simulink model "SF105A_MotCurrRegVltgLimr"  (R2013b)
settings: Solver=FixedStepDiscrete  SolverMode=SingleTasking  StartTime=0.0  StopTime=1  FixedStep=0.00025  RelTol=1e-3
undefined symbols (not defined in the file): ARCHGLBPRM_2OVERSQRT3_ULS_F32, ARCHGLBPRM_2PI_ULS_F32, BRDGVLTGHILIM_VOLT_F32, ELECGLBPRM_PWMPERDNOMX2_SEC_F32, F32TOU16OVR2PI_ULS_F32, MotCurrRegCfgCurrLoopSecOrderTrfFctEna, MotCurrRegCfgMotRVirtDax, MotCurrRegCfgMotRVirtQax, MotCurrRegVltgLimrCurrLoaScarSlewRate, MotCurrRegVltgLimrDaxAntiWdupCoeff, MotCurrRegVltgLimrDualEcuLoaScarSlewRate, MotCurrRegVltgLimrIvtrLoaScarSlewRate, MotCurrRegVltgLimrMotCurrPredEna, MotCurrRegVltgLimrMotCurrPredTi, MotCurrRegVltgLimrMotCurrQaxRefMdfnRplEna, MotCurrRegVltgLimrMotVltgBrdgFilEna, MotCurrRegVltgLimrMotVltgDaxIntglHiLim, MotCurrRegVltgLimrMotVltgDaxIntglLoLim, MotCurrRegVltgLimrMotVltgQaxFfFilEna, MotCurrRegVltgLimrMotVltgQaxIntglHiLim, MotCurrRegVltgLimrMotVltgQaxIntglLoLim, MotCurrRegVltgLimrQaxAntiWdupCoeff, MotCurrRegVltgLimrQaxAntiWdupScagDi, MotRefMdlFbCtrlDi, MotRefMdlIvtrDeadTiBrdgVltgSca, SysSt1, ZERO_VOLT_F32
libraries: NxtrLim x15, Fil x4, simulink x3, NxtrMax x2, NxtrMin x2
(part 1 of 5)
settings Model: Creator=qzwc4r  LastModifiedBy=DZ1YRM
settings SolverCC: AutoInsertRateTranBlk=on  InsertRTBMode=Always
settings DataIOCC: LimitDataPoints=off  SaveFormat=Structure  ReturnWorkspaceOutputs=on
settings OptimizationCC: BlockReduction=off  InlineParams=on  ZeroExternalMemoryAtStartup=off  ZeroInternalMemoryAtStartup=off  OptimizeModelRefInitCode=on  LifeSpan=1
settings DebuggingCC: SignalInfNanChecking=error  SignalRangeChecking=warning  UnderspecifiedInitializationDetection=Simplified  SolverPrmCheckMsg=error  InheritedTsInSrcMsg=error  DiscreteInheritContinuousMsg=error  SingleTaskRateTransMsg=error  TasksWithSamePriorityMsg=error  SigSpecEnsureSampleTimeMsg=error  CheckMatrixSingularityMsg=error  ParameterUnderflowMsg=error  ParameterPrecisionLossMsg=error  ParameterTunabilityLossMsg=error  FixptConstUnderflowMsg=warning  FixptConstOverflowMsg=warning  VectorMatrixConversionMsg=error  SignalLabelMismatchMsg=error  UnconnectedInputMsg=error  UnconnectedOutputMsg=error  UnconnectedLineMsg=error  SFcnCompatibilityMsg=error  UniqueDataStoreMsg=warning  BusObjectLabelMismatch=error  RootOutportRequireBusObject=error  AssertControl=DisableAll  ModelReferenceIOMsg=error  ModelReferenceVersionMismatchMessage=warning  ModelReferenceIOMismatchMessage=error  ModelReferenceCSMismatchMessage=warning  ModelReferenceDataLoggingMessage=error  StateNameClashWarn=warning  StrictBusMsg=ErrorOnBusTreatedAsVector  NonBusSignalsTreatedAsBus=error  SFUnexpectedBacktrackingDiag=error  SFInvalidInputDataAccessInChartInitDiag=error  SFNoUnconditionalDefaultTransitionDiag=error  SFTransitionOutsideNaturalParentDiag=error  SFUnconditionalTransitionShadowingDiag=error  SFUndirectedBroadcastEventsDiag=error
settings ModelReferenceCC: ModelReferenceNumInstancesAllowed=Single
settings RTWCC: SystemTargetFile=autosar.tlc  GenCodeOnly=on  TemplateMakefile=ert_default_tmf  Description=AUTOSAR  GenerateReport=on  ProcessScript=autosar_make_rtw_hook  LaunchReport=on
settings CodeAppCC: GenerateComments=off  IgnoreCustomStorageClasses=off  CustomSymbolStrType=$N$R$M  CustomSymbolStrBlkIO=$N$M  SimulinkBlockComments=off
settings STFCustomTargetCC: ParMdlRefBuildCompliant=on  CompOptLevelCompliant=on  IncludeMdlTerminateFcn=off  CombineOutputUpdateFcns=on  SuppressErrorStatus=on  ERTFirstTimeCompliant=on  ERTCustomFileBanners=on  SupportNonFinite=off  SupportComplex=off  SupportContinuousTime=off  SupportNonInlinedSFcns=off  MATLABClassNameForMDSCustomization=Simulink.SoftwareTarget.ERTCustomization  AutosarCompliant=on  GRTInterface=off  SystemTargetFile=autosar.tlc
settings ERTTargetCC: CodeReplacementLibrary=ANSI_C  ConcurrentExecutionCompliant=off  IncludeMdlTerminateFcn=off  SuppressErrorStatus=on  SupportNonFinite=off  SupportComplex=off  ModelStepFunctionPrototypeControlCompliant=off  CPPClassGenCompliant=off  AutosarCompliant=on  InlinedParameterPlacement=NonHierarchical  ERTCustomFileTemplate=example_file_process.tlc  EnableUserReplacementTypes=on

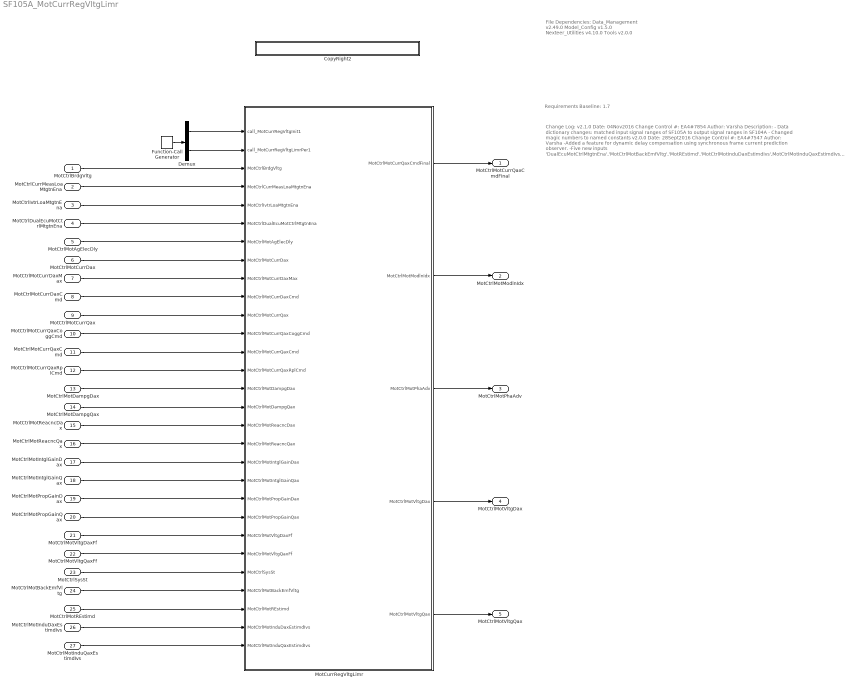
== system SF105A_MotCurrRegVltgLimr ==
  note: File Dependencies:
      |
      | Data_Management v2.49.0
      | Model_Config v1.5.0
      | Nexteer_Utilities v4.10.0
      | Tools v2.0.0
  note: Requirements Baseline: 1.7
  note: Change Log:
      |
      | v2.1.0
      | Date: 04Nov2016
      | Change Control #: EA4#7854
      | Author: Varsha
      | Description:
      | - Data dictionary changes: matched input signal ranges of SF105A to output signal ranges in SF104A
      | - Changed magic numbers to named constants
      |
      |
      | v2.0.0
      | Date: 28Sept2016
      | Change Control #: EA4#7547
      | Author: Varsha
      | -Added a feature for dynamic delay compensation using synchronous frame current prediction observer.
      | -Five new inputs 'DualEcuMotCtrlMtgtnEna','MotCtrlMotBackEmfVltg','MotREstimd','MotCtrlMotInduDaxEstimdIvs',MotCtrlMotInduQaxEstimdIvs
      | have been added to model and data dictionary.
      | -Two new calibrations 'MotCurrRegVltgLimrMotCurrPredEna','MotCurrRegVltgLimrMotCurrPredTi' have been added.
      | -A new constant 'ARCHGLBPRM_2OVERSQRT3_ULS_F32' has been added.
      | -Two per-instance memory blocks 'MotCtrlMotVltgQaxPrev' and 'MotCtrlMotVltgDaxPrev' have been added
      | -Updated design for switching to feedforward control operation during application faulted conditions where single ECU is operational
      |
      | v1.8.0
      | Date: 13Sep2016
      | Change Control #: EA4#7472
      | Author: Siva
      | Description:
      | - Used latest Low Pass filter Initialization blocks.
      |
      | v1.7.0
      | Date: 26Aug2016
      | Change Control #: EA4#7221
      | Author: Siva
      | Description:
      | - Updated Data type conversion block used for calculating Phase Advance from "f32 to u0p16" to "f32 to u16p0"
      |   as the value is converted to "u0p16" upfront using "F32TOU16OVR2PI_ULS_F32" constant.
      |
      |
      | v1.6.0
      | Date: 15Aug2016
      | Change Control #: EA4#6632
      | Author: Siva
      | Description:
      | - Two new constants 'MOTVLTGDQAXLOLIM_VOLT_F32' & 'MOTVLTGDQAXHILIM_VOLT_F32' have been added to
      |   model and Data Dictionary with values -26.5V and +26.5 V respectively for range limiting 'MotCtrlMotVltgDax'
      |   and 'MotCtrlMotVltgQax'.
      | - Two new constants 'PHAADVLOLIM_MOTREV_F32' & 'PHAADVHILIM_MOTREV_F32' have been added to
      |   model and Data Dictionary with values 0 and 65535 respectively for range limiting 'Phase Advance' floating point value.
      | - Updated 'F32TOU16OVR2PI_ULS_F32' constant Value to '10430.21921' instead of '10430.194'.
      | - Removed Saturation limits for 'MotCtrlMotPhaAdv' output signal and added a new Data Type conversion block to
      |   convert float value to u0p16 value.
      | - Removed 'MOTPHAADVHILIM_MOTREV_U0P16' & 'MOTPHAADVLOLIM_MOTREV_U0P16' from Data Dictionary.
      |
      |
      | v1.5.1
      | Date: 29April2016
      | Change Control #: EA4#5367
      | Author: Siva
      | Description:
      | - HIghlighted only those blocks related to v1.5.0.
      |
      |
      | v1.5.0
      | Date: 29April2016
      | Change Control #: EA4#5367
      | Author: Siva
      | Description:
      | - Input signal name changed from 'MotCtrlMotCurrLoaMtgtnEna' to 'MotCtrlCurrMeasLoaMtgtnEna'.
      | - Ranges of calibrations 'MotCurrRegVltgLimrDaxAntiWdupCoeff ' and 'MotCurrRegVltgLimrQaxAntiWdupCoeff'
      |    were updated to -1 & 1 instead of -25 & 25.
      |
      |
      | v1.4.0
      | Date: 04April2015
      | Change Control #: EA4#4493
      | Author: Fei Yuan
      | Description:
      | - Add selectable location for multiply of q axis inverse ratio (multiply by Iq reference , or
      |   multiply by the summation of the Iq reference and Iq ripple and Iq cogging signals).
      | - Add signal range limit on integrator state viriables for q and d axis paths.
      | - Add singal range limit on current reference command per defined signal ranges.
      | - Add signed calibratable integrator state vairable limits.
      |
      | v1.3.0
      | Date: 20November2015
      | Change Control #: EA4#2392
      | Author: Fei Yuan
      | Description:
      | - Add range limiters to outputs
      | - Update the Dependencies in the Data Dict
      | - Correct some keywords based on the keyword list.
      |
      | v1.2.0
      | Date: 05June2015
      | Change Control #: EA4#630
      | DRW: P. Lefler
      | Description:
      | - Fixes to calibration names and data types in DataDict file and Dependencies file.
      |
      | v1.1.0
      | Date: 26May2015
      | Change Control #: EA4#630
      | DRW: P. Lefler
      | Description:
      | - Changes for algorithm optimization, output datatype change, and added requirements links
      |
      | v1.0.0
      | Date: 07May2015
      | Change Control #: EA4#297
      | DRW: P. Lefler
      | Description:
      | - Initial Release
  MotCtrlBrdgVltg : Inport  RequirementInfo={} %GIDa_8e46ce2a_919a_4506_8698_295a99460b12
  MotCtrlCurrMeasLoaMtgtnEna : Inport  RequirementInfo={} %GIDa_af8bb34f_046c_46e7_bd5e_44b54be0502c  Port=2
  MotCtrlIvtrLoaMtgtnEna : Inport  RequirementInfo={} %GIDa_3adfcd90_572b_4e35_8cfd_3c676c239ace  Port=3
  MotCtrlDualEcuMotCtrlMtgtnEna : Inport  RequirementInfo={} %GIDa_4618ed0f_79cf_46df_8a31_52c1690ffb8d  Port=4
  MotCtrlMotAgElecDly : Inport  RequirementInfo={} %GIDa_d64dbb74_7a6c_48e8_b5fd_fb09433ca9f0  Port=5
  MotCtrlMotCurrDax : Inport  RequirementInfo={} %GIDa_e7d34867_bb71_42aa_ae81_73d704cf4016  Port=6
  MotCtrlMotCurrDaxMax : Inport  RequirementInfo={} %GIDa_95b74bd1_5092_49ca_9d39_f9500bf46caa  Port=7
  MotCtrlMotCurrDaxCmd : Inport  RequirementInfo={} %GIDa_68535612_aa98_4b73_9e8e_7c7f66964449  Port=8
  MotCtrlMotCurrQax : Inport  RequirementInfo={} %GIDa_c3d95f7e_4c05_48b0_9da3_bf75894c8661  Port=9
  MotCtrlMotCurrQaxCoggCmd : Inport  RequirementInfo={} %GIDa_d050ecd7_013f_4c96_959a_36eb92ce70ab  Port=10
  MotCtrlMotCurrQaxCmd : Inport  RequirementInfo={} %GIDa_168a24af_4211_4955_a405_77a28ee6b1d8  Port=11
  MotCtrlMotCurrQaxRplCmd : Inport  RequirementInfo={} %GIDa_80f96bb1_811c_4e5c_9c99_d0a2b6d1b546  Port=12
  MotCtrlMotDampgDax : Inport  RequirementInfo={} %GIDa_b4263008_b2fe_479b_ab1a_58326cb85cc1  Port=13
  MotCtrlMotDampgQax : Inport  RequirementInfo={} %GIDa_a343ed71_2ec5_45b3_affe_06b72ae41368  Port=14
  MotCtrlMotReacncDax : Inport  RequirementInfo={} %GIDa_7ae76b1f_2e5a_4874_a1b1_4f7855b8eb50  Port=15
  MotCtrlMotReacncQax : Inport  RequirementInfo={} %GIDa_449f7c36_82cf_4545_8870_73d8e079324d  Port=16
  MotCtrlMotIntglGainDax : Inport  RequirementInfo={} %GIDa_cacd28ef_1570_42d0_8667_de1d5331061d  Port=17
  MotCtrlMotIntglGainQax : Inport  RequirementInfo={} %GIDa_7b09e5f0_cde6_4194_ac39_427519b5ea3c  Port=18
  MotCtrlMotPropGainDax : Inport  RequirementInfo={} %GIDa_722006e4_8def_4c05_955c_20c680c4187a  Port=19
  MotCtrlMotPropGainQax : Inport  RequirementInfo={} %GIDa_be3d4734_242e_476b_ad0b_e25551c24b0a  Port=20
  MotCtrlMotVltgDaxFf : Inport  RequirementInfo={} %GIDa_4efd4844_8ea8_4406_ae94_9804efa9585d  Port=21
  MotCtrlMotVltgQaxFf : Inport  RequirementInfo={} %GIDa_ea442c22_c1cc_4f4a_ada8_81dc7a709cab  Port=22
  MotCtrlSysSt : Inport  RequirementInfo={} %GIDa_be26f1e0_3c0f_4120_aff8_be82e7f083a9  Port=23  OutDataTypeStr=Enum: SysSt1
  MotCtrlMotBackEmfVltg : Inport  RequirementInfo={} %GIDa_f2f564dd_6c3b_46de_9e0e_fc636de52404  Port=24
  MotCtrlMotREstimd : Inport  RequirementInfo={} %GIDa_073120b6_1808_4f14_9c51_29be78d8addc  Port=25
  MotCtrlMotInduDaxEstimdIvs : Inport  RequirementInfo={} %GIDa_a3f48710_1a7a_486c_93c5_3361410e9b98  Port=26
  MotCtrlMotInduQaxEstimdIvs : Inport  RequirementInfo={} %GIDa_79e37907_edf5_439e_bcd8_a58d2ffa50f0  Port=27
  CopyRight2 : Subsystem  Description=|  mask(Copyright Information){none=on}
      | Copyright info block.                                               
      |                                                                     
      | Place copyright information at the top of every subsystem in design.
      mask prompts: none "No parameters"
      mask help: Place copyright information at the top of every subsystem in design.
      mask Display:
      | NxtrConf = 'Nexteer Confidential';
      | 
      | sys = bdroot; %handle for the current model ("system")
      | first = get_param(sys,'Created');
      | if(isempty(first))
      |     first = datestr(now,'yyyy');
      | else
      |     first = first(end-3:end);  %year is last four digits
      | end
      | 
      | last = get_param(sys,'LastModifiedDate');
      | if isempty(last)
      |     last = datestr(now,'yyyy');
      | else
      |     last = last(end-3:end);
      | end
      | 
      | if strcmp(first,last)
      |     fprintf('%s -- Copyright %s Nexteer',NxtrConf,first)
      | else
      |     fprintf('%s -- %s%s- %s Nexteer',NxtrConf,char(169),first,last)
      | end
  Demux : Demux  RequirementInfo={} %GIDa_92189e2f_23ba_494e_b896_c9965fe7d6cd  Outputs=2
  Function-Call Generator : simulink/Ports & Subsystems/Function-Call Generator  RequirementInfo={} %GIDa_d141ba28_1e0a_463b_8f2d_81283afd4db2  sample_time=0.00025  numberOfIterations=1
  MotCurrRegVltgLimr : Subsystem  RequirementInfo={} %GIDa_4642b19e_a30e_4e3c_ab8d_d9e3c3d7ba7b
  MotCtrlMotCurrQaxCmdFinal : Outport  RequirementInfo={} %GIDa_781c28aa_2acd_4b18_9286_344174e8cff2
  MotCtrlMotModlnIdx : Outport  RequirementInfo={} %GIDa_fa51f03d_b9dc_4a13_83b1_4b78852e742e  Port=2
  MotCtrlMotPhaAdv : Outport  RequirementInfo={} %GIDa_ace5b006_310e_4410_94f4_88e59214d43e  Port=3
  MotCtrlMotVltgDax : Outport  RequirementInfo={} %GIDa_04c00acb_66a3_42fd_8198_77a8e17ba56b  Port=4
  MotCtrlMotVltgQax : Outport  RequirementInfo={} %GIDa_039e9d87_d2c8_4e76_ac69_f28813825f03  Port=5
  wires:
  Function-Call Generator/1 -> Demux/1
  Demux/2 -> MotCurrRegVltgLimr/2(call_MotCurrRegVltgLimrPer1)
  Demux/1 -> MotCurrRegVltgLimr/1(call_MotCurrRegVltgInit1)
  MotCtrlBrdgVltg/1 -> MotCurrRegVltgLimr/3(MotCtrlBrdgVltg)
  MotCtrlCurrMeasLoaMtgtnEna/1 -> MotCurrRegVltgLimr/4(MotCtrlCurrMeasLoaMtgtnEna)
  MotCtrlIvtrLoaMtgtnEna/1 -> MotCurrRegVltgLimr/5(MotCtrlIvtrLoaMtgtnEna)
  MotCtrlMotAgElecDly/1 -> MotCurrRegVltgLimr/7(MotCtrlMotAgElecDly)
  MotCtrlMotCurrDax/1 -> MotCurrRegVltgLimr/8(MotCtrlMotCurrDax)
  MotCtrlMotCurrDaxMax/1 -> MotCurrRegVltgLimr/9(MotCtrlMotCurrDaxMax)
  MotCtrlMotCurrDaxCmd/1 -> MotCurrRegVltgLimr/10(MotCtrlMotCurrDaxCmd)
  MotCtrlMotCurrQax/1 -> MotCurrRegVltgLimr/11(MotCtrlMotCurrQax)
  MotCtrlMotCurrQaxCoggCmd/1 -> MotCurrRegVltgLimr/12(MotCtrlMotCurrQaxCoggCmd)
  MotCtrlMotCurrQaxCmd/1 -> MotCurrRegVltgLimr/13(MotCtrlMotCurrQaxCmd)
  MotCtrlMotCurrQaxRplCmd/1 -> MotCurrRegVltgLimr/14(MotCtrlMotCurrQaxRplCmd)
  MotCtrlMotDampgDax/1 -> MotCurrRegVltgLimr/15(MotCtrlMotDampgDax)
  MotCtrlMotDampgQax/1 -> MotCurrRegVltgLimr/16(MotCtrlMotDampgQax)
  MotCtrlMotReacncDax/1 -> MotCurrRegVltgLimr/17(MotCtrlMotReacncDax)
  MotCtrlMotReacncQax/1 -> MotCurrRegVltgLimr/18(MotCtrlMotReacncQax)
  MotCtrlMotIntglGainDax/1 -> MotCurrRegVltgLimr/19(MotCtrlMotIntglGainDax)
  MotCtrlMotIntglGainQax/1 -> MotCurrRegVltgLimr/20(MotCtrlMotIntglGainQax)
  MotCtrlMotPropGainDax/1 -> MotCurrRegVltgLimr/21(MotCtrlMotPropGainDax)
  MotCtrlMotPropGainQax/1 -> MotCurrRegVltgLimr/22(MotCtrlMotPropGainQax)
  MotCtrlMotVltgDaxFf/1 -> MotCurrRegVltgLimr/23(MotCtrlMotVltgDaxFf)
  MotCtrlMotVltgQaxFf/1 -> MotCurrRegVltgLimr/24(MotCtrlMotVltgQaxFf)
  MotCtrlSysSt/1 -> MotCurrRegVltgLimr/25(MotCtrlSysSt)
  MotCurrRegVltgLimr/2(MotCtrlMotModlnIdx) -> MotCtrlMotModlnIdx/1
  MotCurrRegVltgLimr/3(MotCtrlMotPhaAdv) -> MotCtrlMotPhaAdv/1
  MotCurrRegVltgLimr/1(MotCtrlMotCurrQaxCmdFinal) -> MotCtrlMotCurrQaxCmdFinal/1
  MotCurrRegVltgLimr/4(MotCtrlMotVltgDax) -> MotCtrlMotVltgDax/1
  MotCurrRegVltgLimr/5(MotCtrlMotVltgQax) -> MotCtrlMotVltgQax/1
  MotCtrlMotBackEmfVltg/1 -> MotCurrRegVltgLimr/26(MotCtrlMotBackEmfVltg)
  MotCtrlMotREstimd/1 -> MotCurrRegVltgLimr/27(MotCtrlMotREstimd)
  MotCtrlMotInduDaxEstimdIvs/1 -> MotCurrRegVltgLimr/28(MotCtrlMotInduDaxEstimdIvs)
  MotCtrlMotInduQaxEstimdIvs/1 -> MotCurrRegVltgLimr/29(MotCtrlMotInduQaxEstimdIvs)
  MotCtrlDualEcuMotCtrlMtgtnEna/1 -> MotCurrRegVltgLimr/6(MotCtrlDualEcuMotCtrlMtgtnEna)

== system SF105A_MotCurrRegVltgLimr/CopyRight2 ==

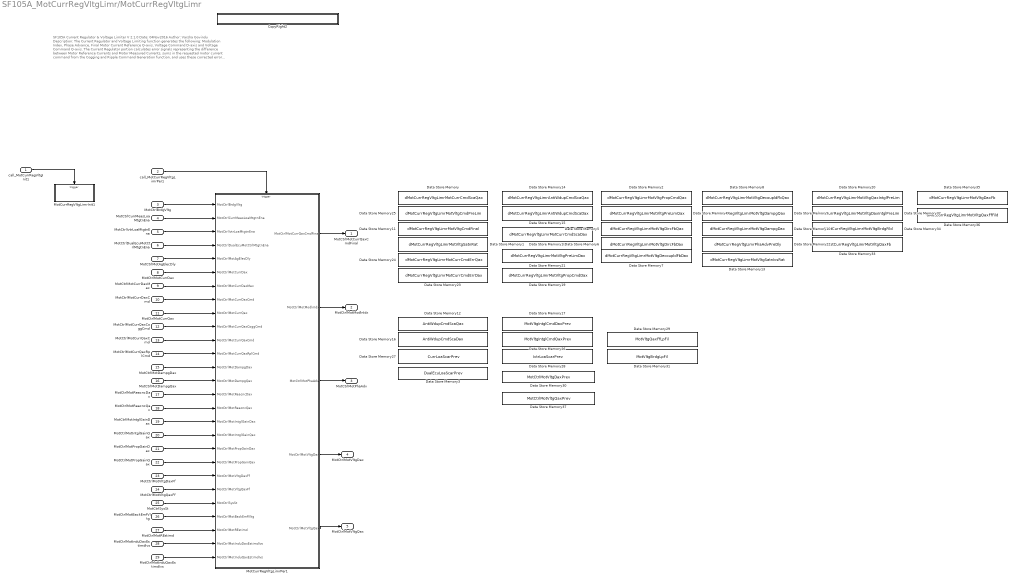
== system SF105A_MotCurrRegVltgLimr/MotCurrRegVltgLimr ==
  note: SF105A Current Regulator & Voltage Limiter
      | V 2.1.0
      | Date: 04Nov2016
      | Author: Varsha Govindu
      | Description: The Current Regulator and Voltage Limiting function generates the following: Modulation Index, Phase Advance, Final Motor Current Reference Q-axis,
      | Voltage Command D-axis and Voltage Command Q-axis.
      | The Current Regulator portion calculates error signals representing the difference between Motor Reference Currents and Motor Measured Currents, sums in the
      | requested motor current command from the Cogging and Ripple Command Generation function, and uses these corrected error signals modified by proportional and
      | integral gains to generate a portion of the voltage command to the motor.  The Current Regulator also applies separate gains to the measured motor currents to
      | generate an additional portion of the voltage command.  The Feedforward Voltages from the Motor Reference model are added to the other two portions to generate
      | the total requested motor voltage command.
      | The Voltage Limiting portion of the function compares the total requested motor voltage command to the total voltage available at the inverter, and implements a limiting
      | and reference command correcting function in order to prevent windup of Current Regulator states and improve reference command tracking.
  call_MotCurrRegVltgInit1 : Inport
  call_MotCurrRegVltgLimrPer1 : Inport  Port=2
  MotCtrlBrdgVltg : Inport  RequirementInfo={'linktype_rmi_doors' '0000bb44 (/E-STEER Core/SubSystem Specifications/Application Functions/SF99/SF105A Current Regulator and Voltage Limiter)' '#SF105A_58' 'true' 'REQ: SF105A_58' '' ; 'linktype_rmi_doors' '0000bb44 (/E-STEER Core/SubSystem Specifications/Application Functions/SF99/SF105A Current Regulator and Voltage Limiter)' '#SF105A_166' 'true' 'REQ: SF105A_166' '' } %GIDa_606dfb72_cb0e_4bf4_a448_cf2d667aea26  Port=3
  MotCtrlCurrMeasLoaMtgtnEna : Inport  RequirementInfo={'linktype_rmi_doors' '0000bb44 (/E-STEER Core/SubSystem Specifications/Application Functions/SF99/SF105A Current Regulator and Voltage Limiter)' '#SF105A_59' 'true' 'REQ: SF105A_59' '' ; 'linktype_rmi_doors' '0000bb44 (/E-STEER Core/SubSystem Specifications/Application Functions/SF99/SF105A Current Regulator and Voltage Limiter)' '#SF105A_168' 'true' 'REQ: SF105A_168' '' } %GIDa_d06f39e9_eb60_46fa_8d46_638325da2097  Port=4
  MotCtrlIvtrLoaMtgtnEna : Inport  RequirementInfo={'linktype_rmi_doors' '0000bb44 (/E-STEER Core/SubSystem Specifications/Application Functions/SF99/SF105A Current Regulator and Voltage Limiter)' '#SF105A_153' 'true' 'REQ: SF105A_153' '' ; 'linktype_rmi_doors' '0000bb44 (/E-STEER Core/SubSystem Specifications/Application Functions/SF99/SF105A Current Regulator and Voltage Limiter)' '#SF105A_168' 'true' 'REQ: SF105A_168' '' } %GIDa_81420cc2_8e05_4f74_9716_a5648030ffcb  Port=5
  MotCtrlDualEcuMotCtrlMtgtnEna : Inport  RequirementInfo={'linktype_rmi_doors' '0000bb44 (/E-STEER Core/SubSystem Specifications/Application Functions/SF99/SF105A Current Regulator and Voltage Limiter)' '#SF105A_199' 'true' 'REQ: SF105A_199' '' } %GIDa_f8a239b4_df34_4f4d_ae99_1298116ecc14  Port=6
  MotCtrlMotAgElecDly : Inport  RequirementInfo={'linktype_rmi_doors' '0000bb44 (/E-STEER Core/SubSystem Specifications/Application Functions/SF99/SF105A Current Regulator and Voltage Limiter)' '#SF105A_46' 'true' 'REQ: SF105A_46' '' } %GIDa_86188211_fab5_49f2_9b91_c05f705e3c63  Port=7
  MotCtrlMotCurrDax : Inport  RequirementInfo={'linktype_rmi_doors' '0000bb44 (/E-STEER Core/SubSystem Specifications/Application Functions/SF99/SF105A Current Regulator and Voltage Limiter)' '#SF105A_57' 'true' 'REQ: SF105A_57' '' } %GIDa_0b9d98be_f12b_4977_b4e0_ba90ca28ad52  Port=8
  MotCtrlMotCurrDaxMax : Inport  RequirementInfo={'linktype_rmi_doors' '0000bb44 (/E-STEER Core/SubSystem Specifications/Application Functions/SF99/SF105A Current Regulator and Voltage Limiter)' '#SF105A_53' 'true' 'REQ: SF105A_53' '' } %GIDa_6012c004_0bcf_42a3_ab54_1ad4e16fdcd8  Port=9
  MotCtrlMotCurrDaxCmd : Inport  RequirementInfo={'linktype_rmi_doors' '0000bb44 (/E-STEER Core/SubSystem Specifications/Application Functions/SF99/SF105A Current Regulator and Voltage Limiter)' '#SF105A_38' 'true' 'REQ: SF105A_38' '' } %GIDa_3c8cfcc2_1716_43e3_a5f4_74f0cc4785f3  Port=10
  MotCtrlMotCurrQax : Inport  RequirementInfo={'linktype_rmi_doors' '0000bb44 (/E-STEER Core/SubSystem Specifications/Application Functions/SF99/SF105A Current Regulator and Voltage Limiter)' '#SF105A_56' 'true' 'REQ: SF105A_56' '' } %GIDa_f2105923_8b5d_4c38_b5d7_d8944874b87d  Port=11
  MotCtrlMotCurrQaxCoggCmd : Inport  RequirementInfo={'linktype_rmi_doors' '0000bb44 (/E-STEER Core/SubSystem Specifications/Application Functions/SF99/SF105A Current Regulator and Voltage Limiter)' '#SF105A_47' 'true' 'REQ: SF105A_47' '' } %GIDa_5eb15454_dd57_4a66_beac_3c42276a2f51  Port=12
  MotCtrlMotCurrQaxCmd : Inport  RequirementInfo={'linktype_rmi_doors' '0000bb44 (/E-STEER Core/SubSystem Specifications/Application Functions/SF99/SF105A Current Regulator and Voltage Limiter)' '#SF105A_27' 'true' 'REQ: SF105A_27' '' } %GIDa_00ed98c3_1b47_4f14_b89e_6bdb9443e2b5  Port=13
  MotCtrlMotCurrQaxRplCmd : Inport  RequirementInfo={'linktype_rmi_doors' '0000bb44 (/E-STEER Core/SubSystem Specifications/Application Functions/SF99/SF105A Current Regulator and Voltage Limiter)' '#SF105A_48' 'true' 'REQ: SF105A_48' '' } %GIDa_164b68d2_17d4_417d_9d13_ce78fec31a24  Port=14
  MotCtrlMotDampgDax : Inport  RequirementInfo={'linktype_rmi_doors' '0000bb44 (/E-STEER Core/SubSystem Specifications/Application Functions/SF99/SF105A Current Regulator and Voltage Limiter)' '#SF105A_51' 'true' 'REQ: SF105A_51' '' } %GIDa_d80b900b_5b17_49e7_a0fb_1c642e6dbeab  Port=15
  MotCtrlMotDampgQax : Inport  RequirementInfo={'linktype_rmi_doors' '0000bb44 (/E-STEER Core/SubSystem Specifications/Application Functions/SF99/SF105A Current Regulator and Voltage Limiter)' '#SF105A_52' 'true' 'REQ: SF105A_52' '' } %GIDa_135f8750_4a7b_4123_b230_75ae30cebc17  Port=16
  MotCtrlMotReacncDax : Inport  RequirementInfo="{'linktype_rmi_doors' '0000bb44 (/E-STEER Core/SubSystem Specifications/Application Functions/SF99/SF105A Current Regulator and Voltage Limiter)' '#SF105A_200' 'true' 'REQ:  SF105A_200' '' } %GIDa_6cdc6bde_4ecf_4a2e_aa1c_ab6a1c2bbfa0"  Port=17
  MotCtrlMotReacncQax : Inport  RequirementInfo="{'linktype_rmi_doors' '0000bb44 (/E-STEER Core/SubSystem Specifications/Application Functions/SF99/SF105A Current Regulator and Voltage Limiter)' '#SF105A_201' 'true' 'REQ:  SF105A_201' '' } %GIDa_d20b8c12_f6fe_452e_895e_2c4818144197"  Port=18
  MotCtrlMotIntglGainDax : Inport  RequirementInfo={'linktype_rmi_doors' '0000bb44 (/E-STEER Core/SubSystem Specifications/Application Functions/SF99/SF105A Current Regulator and Voltage Limiter)' '#SF105A_43' 'true' 'REQ: SF105A_43' '' } %GIDa_ff2cdd4f_5724_43e1_9917_ebab471fd46c  Port=19
  MotCtrlMotIntglGainQax : Inport  RequirementInfo={'linktype_rmi_doors' '0000bb44 (/E-STEER Core/SubSystem Specifications/Application Functions/SF99/SF105A Current Regulator and Voltage Limiter)' '#SF105A_41' 'true' 'REQ: SF105A_41' '' } %GIDa_98726177_a4e0_47cc_b58f_31ebce95769b  Port=20
  MotCtrlMotPropGainDax : Inport  RequirementInfo={'linktype_rmi_doors' '0000bb44 (/E-STEER Core/SubSystem Specifications/Application Functions/SF99/SF105A Current Regulator and Voltage Limiter)' '#SF105A_42' 'true' 'REQ: SF105A_42' '' } %GIDa_6535565c_4545_4794_bf38_f6d900ca01ae  Port=21
  MotCtrlMotPropGainQax : Inport  RequirementInfo={'linktype_rmi_doors' '0000bb44 (/E-STEER Core/SubSystem Specifications/Application Functions/SF99/SF105A Current Regulator and Voltage Limiter)' '#SF105A_40' 'true' 'REQ: SF105A_40' '' } %GIDa_b7091800_b160_4923_a856_7876a39339aa  Port=22
  MotCtrlMotVltgDaxFf : Inport  RequirementInfo={'linktype_rmi_doors' '0000bb44 (/E-STEER Core/SubSystem Specifications/Application Functions/SF99/SF105A Current Regulator and Voltage Limiter)' '#SF105A_45' 'true' 'REQ: SF105A_45' '' } %GIDa_535439cb_455e_4dfa_bd22_9f04eb631c24  Port=23
  MotCtrlMotVltgQaxFf : Inport  RequirementInfo={'linktype_rmi_doors' '0000bb44 (/E-STEER Core/SubSystem Specifications/Application Functions/SF99/SF105A Current Regulator and Voltage Limiter)' '#SF105A_44' 'true' 'REQ: SF105A_44' '' } %GIDa_090e0805_6815_412d_9c46_56beeea73767  Port=24
  MotCtrlSysSt : Inport  RequirementInfo={'linktype_rmi_doors' '0000bb44 (/E-STEER Core/SubSystem Specifications/Application Functions/SF99/SF105A Current Regulator and Voltage Limiter)' '#SF105A_161' 'true' 'REQ: SF105A_161' '' ; 'linktype_rmi_doors' '0000bb44 (/E-STEER Core/SubSystem Specifications/Application Functions/SF99/SF105A Current Regulator and Voltage Limiter)' '#SF105A_169' 'true' 'REQ: SF105A_169' '' } %GIDa_5200f575_fdfb_4c92_b49b_ed00ed8ebeb1  Port=25  OutDataTypeStr=Enum: SysSt1
  MotCtrlMotBackEmfVltg : Inport  RequirementInfo={'linktype_rmi_doors' '0000bb44 (/E-STEER Core/SubSystem Specifications/Application Functions/SF99/SF105A Current Regulator and Voltage Limiter)' '#SF105A_202' 'true' 'REQ: SF105A_202' '' } %GIDa_ea253e08_4b49_4115_9be9_6e902e8e4a32  Port=26
  MotCtrlMotREstimd : Inport  RequirementInfo={'linktype_rmi_doors' '0000bb44 (/E-STEER Core/SubSystem Specifications/Application Functions/SF99/SF105A Current Regulator and Voltage Limiter)' '#SF105A_203' 'true' 'REQ: SF105A_203' '' } %GIDa_7d65b8bc_43bd_46b9_9afb_21630165c386  Port=27
  MotCtrlMotInduDaxEstimdIvs : Inport  RequirementInfo={'linktype_rmi_doors' '0000bb44 (/E-STEER Core/SubSystem Specifications/Application Functions/SF99/SF105A Current Regulator and Voltage Limiter)' '#SF105A_204' 'true' 'REQ: SF105A_204' '' } %GIDa_9848b0b3_667c_4e17_a13b_b834f23d5e07  Port=28
  MotCtrlMotInduQaxEstimdIvs : Inport  RequirementInfo={'linktype_rmi_doors' '0000bb44 (/E-STEER Core/SubSystem Specifications/Application Functions/SF99/SF105A Current Regulator and Voltage Limiter)' '#SF105A_205' 'true' 'REQ: SF105A_205' '' } %GIDa_051361da_ee1e_4770_b948_9b22e6e78646  Port=29
  CopyRight2 : Subsystem  Description=|  mask(Copyright Information){none=on}
      | Copyright info block.                                               
      |                                                                     
      | Place copyright information at the top of every subsystem in design.
      mask prompts: none "No parameters"
      mask help: Place copyright information at the top of every subsystem in design.
      mask Display:
      | NxtrConf = 'Nexteer Confidential';
      | 
      | sys = bdroot; %handle for the current model ("system")
      | first = get_param(sys,'Created');
      | if(isempty(first))
      |     first = datestr(now,'yyyy');
      | else
      |     first = first(end-3:end);  %year is last four digits
      | end
      | 
      | last = get_param(sys,'LastModifiedDate');
      | if isempty(last)
      |     last = datestr(now,'yyyy');
      | else
      |     last = last(end-3:end);
      | end
      | 
      | if strcmp(first,last)
      |     fprintf('%s -- Copyright %s Nexteer',NxtrConf,first)
      | else
      |     fprintf('%s -- %s%s- %s Nexteer',NxtrConf,char(169),first,last)
      | end
  Data Store Memory : DataStoreMemory  DataStoreName=dMotCurrRegVltgLimrMotCurrCmdScaQax  ReadBeforeWriteMsg=warning  WriteAfterWriteMsg=warning  WriteAfterReadMsg=warning  StateMustResolveToSignalObject=on
  Data Store Memory1 : DataStoreMemory  DataStoreName=dMotCurrRegVltgLimrMotVltgSatnRat  ReadBeforeWriteMsg=warning  WriteAfterWriteMsg=warning  WriteAfterReadMsg=warning  StateMustResolveToSignalObject=on
  Data Store Memory10 : DataStoreMemory  DataStoreName=dMotCurrRegVltgLimrMotVltgDampgDax  ReadBeforeWriteMsg=warning  WriteAfterWriteMsg=warning  WriteAfterReadMsg=warning  StateMustResolveToSignalObject=on
  Data Store Memory11 : DataStoreMemory  DataStoreName=dMotCurrRegVltgLimrMotVltgCmdFinal  ReadBeforeWriteMsg=warning  WriteAfterWriteMsg=warning  WriteAfterReadMsg=warning  StateMustResolveToSignalObject=on
  Data Store Memory12 : DataStoreMemory  DataStoreName=AntiWdupCmdScaQax  StateMustResolveToSignalObject=on
  Data Store Memory13 : DataStoreMemory  DataStoreName=dMotCurrRegVltgLimrMotVltgSatnIvsRat  ReadBeforeWriteMsg=warning  WriteAfterWriteMsg=warning  WriteAfterReadMsg=warning  StateMustResolveToSignalObject=on
  Data Store Memory14 : DataStoreMemory  DataStoreName=dMotCurrRegVltgLimrAntiWdupCmdScaQax  ReadBeforeWriteMsg=warning  WriteAfterWriteMsg=warning  WriteAfterReadMsg=warning  StateMustResolveToSignalObject=on
  Data Store Memory15 : DataStoreMemory  DataStoreName=dMotCurrRegVltgLimrAntiWdupCmdScaDax  ReadBeforeWriteMsg=warning  WriteAfterWriteMsg=warning  WriteAfterReadMsg=warning  StateMustResolveToSignalObject=on
  Data Store Memory16 : DataStoreMemory  DataStoreName=AntiWdupCmdScaDax  StateMustResolveToSignalObject=on
  Data Store Memory17 : DataStoreMemory  DataStoreName=MotVltgIntglCmdDaxPrev  StateMustResolveToSignalObject=on
  Data Store Memory18 : DataStoreMemory  DataStoreName=dMotCurrRegVltgLimrMotCurrCmdScaDax  ReadBeforeWriteMsg=warning  WriteAfterWriteMsg=warning  WriteAfterReadMsg=warning  StateMustResolveToSignalObject=on
  Data Store Memory19 : DataStoreMemory  DataStoreName=dMotCurrRegVltgLimrMotVltgPropCmdDax  ReadBeforeWriteMsg=warning  WriteAfterWriteMsg=warning  WriteAfterReadMsg=warning  StateMustResolveToSignalObject=on
  Data Store Memory2 : DataStoreMemory  DataStoreName=dMotCurrRegVltgLimrMotVltgPropCmdQax  ReadBeforeWriteMsg=warning  WriteAfterWriteMsg=warning  WriteAfterReadMsg=warning  StateMustResolveToSignalObject=on
  Data Store Memory20 : DataStoreMemory  DataStoreName=dMotCurrRegVltgLimrMotVltgQaxIntglPreLim  StateMustResolveToSignalObject=on
  Data Store Memory21 : DataStoreMemory  DataStoreName=dMotCurrRegVltgLimrMotVltgPreLimDax  ReadBeforeWriteMsg=warning  WriteAfterWriteMsg=warning  WriteAfterReadMsg=warning  StateMustResolveToSignalObject=on
  Data Store Memory22 : DataStoreMemory  DataStoreName=dMotCurrRegVltgLimrPhaAdvPreDly  ReadBeforeWriteMsg=warning  WriteAfterWriteMsg=warning  WriteAfterReadMsg=warning  StateMustResolveToSignalObject=on
  Data Store Memory23 : DataStoreMemory  DataStoreName=dMotCurrRegVltgLimrMotCurrCmdErrDax  ReadBeforeWriteMsg=warning  WriteAfterWriteMsg=warning  WriteAfterReadMsg=warning  StateMustResolveToSignalObject=on
  Data Store Memory24 : DataStoreMemory  DataStoreName=dMotCurrRegVltgLimrMotCurrCmdErrQax  ReadBeforeWriteMsg=warning  WriteAfterWriteMsg=warning  WriteAfterReadMsg=warning  StateMustResolveToSignalObject=on
  Data Store Memory25 : DataStoreMemory  DataStoreName=dMotCurrRegVltgLimrMotVltgCmdPreLim  ReadBeforeWriteMsg=warning  WriteAfterWriteMsg=warning  WriteAfterReadMsg=warning  StateMustResolveToSignalObject=on
  Data Store Memory26 : DataStoreMemory  RequirementInfo={'linktype_rmi_doors' '0000bb44 (/E-STEER Core/SubSystem Specifications/Application Functions/SF99/SF105A Current Regulator and Voltage Limiter)' '#SF105A_134' 'true' 'REQ: SF105A_134' '' } %GIDa_b9f44faa_5ecd_4ebf_a584_f0271a5711cd  DataStoreName=MotVltgIntglCmdQaxPrev  StateMustResolveToSignalObject=on
  Data Store Memory27 : DataStoreMemory  DataStoreName=CurrLoaScarPrev  StateMustResolveToSignalObject=on
  Data Store Memory28 : DataStoreMemory  DataStoreName=IvtrLoaScarPrev  StateMustResolveToSignalObject=on
  Data Store Memory29 : DataStoreMemory  DataStoreName=MotVltgQaxFfLpFil  InitialValue=[]  OutDataTypeStr=Bus: FilLpRec1  StateMustResolveToSignalObject=on
  Data Store Memory3 : DataStoreMemory  DataStoreName=DualEcuLoaScarPrev  StateMustResolveToSignalObject=on
  Data Store Memory30 : DataStoreMemory  DataStoreName=MotCtrlMotVltgDaxPrev  StateMustResolveToSignalObject=on
  Data Store Memory31 : DataStoreMemory  DataStoreName=MotVltgBrdgLpFil  InitialValue=[]  OutDataTypeStr=Bus: FilLpRec1  StateMustResolveToSignalObject=on
  Data Store Memory32 : DataStoreMemory  DataStoreName=dMotCurrRegVltgLimrMotVltgDaxIntglPreLim  StateMustResolveToSignalObject=on
  Data Store Memory33 : DataStoreMemory  DataStoreName=dMotCurrRegVltgLimrMotVltgQaxFb  ReadBeforeWriteMsg=warning  WriteAfterWriteMsg=warning  WriteAfterReadMsg=warning  StateMustResolveToSignalObject=on
  Data Store Memory34 : DataStoreMemory  DataStoreName=dMotCurrRegVltgLimrMotVltgBrdgFild  StateMustResolveToSignalObject=on
  Data Store Memory35 : DataStoreMemory  DataStoreName=dMotCurrRegVltgLimrMotVltgDaxFb  StateMustResolveToSignalObject=on
  Data Store Memory36 : DataStoreMemory  DataStoreName=dMotCurrRegVltgLimrMotVltgQaxFfFild  StateMustResolveToSignalObject=on
  Data Store Memory37 : DataStoreMemory  DataStoreName=MotCtrlMotVltgQaxPrev  StateMustResolveToSignalObject=on
  Data Store Memory4 : DataStoreMemory  DataStoreName=dMotCurrRegVltgLimrMotVltgPreLimQax  ReadBeforeWriteMsg=warning  WriteAfterWriteMsg=warning  WriteAfterReadMsg=warning  StateMustResolveToSignalObject=on
  Data Store Memory5 : DataStoreMemory  DataStoreName=dMotCurrRegVltgLimrMotVltgDircFbQax  ReadBeforeWriteMsg=warning  WriteAfterWriteMsg=warning  WriteAfterReadMsg=warning  StateMustResolveToSignalObject=on
  Data Store Memory6 : DataStoreMemory  DataStoreName=dMotCurrRegVltgLimrMotVltgDircFbDax  ReadBeforeWriteMsg=warning  WriteAfterWriteMsg=warning  WriteAfterReadMsg=warning  StateMustResolveToSignalObject=on
  Data Store Memory7 : DataStoreMemory  DataStoreName=dMotCurrRegVltgLimrMotVltgDecoupldFbDax  ReadBeforeWriteMsg=warning  WriteAfterWriteMsg=warning  WriteAfterReadMsg=warning  StateMustResolveToSignalObject=on
  Data Store Memory8 : DataStoreMemory  DataStoreName=dMotCurrRegVltgLimrMotVltgDecoupldFbQax  ReadBeforeWriteMsg=warning  WriteAfterWriteMsg=warning  WriteAfterReadMsg=warning  StateMustResolveToSignalObject=on
  Data Store Memory9 : DataStoreMemory  DataStoreName=dMotCurrRegVltgLimrMotVltgDampgQax  ReadBeforeWriteMsg=warning  WriteAfterWriteMsg=warning  WriteAfterReadMsg=warning  StateMustResolveToSignalObject=on
  MotCurrRegVltgLimrInit1 : Subsystem  TreatAsAtomicUnit=on
  MotCurrRegVltgLimrPer1 : Subsystem  TreatAsAtomicUnit=on
  MotCtrlMotCurrQaxCmdFinal : Outport  RequirementInfo={'linktype_rmi_doors' '0000bb44 (/E-STEER Core/SubSystem Specifications/Application Functions/SF99/SF105A Current Regulator and Voltage Limiter)' '#SF105A_61' 'true' 'REQ: SF105A_61' '' } %GIDa_db1260c5_19b4_4bac_ab28_4732f358d49c
  MotCtrlMotModlnIdx : Outport  RequirementInfo={'linktype_rmi_doors' '0000bb44 (/E-STEER Core/SubSystem Specifications/Application Functions/SF99/SF105A Current Regulator and Voltage Limiter)' '#SF105A_28' 'true' 'REQ: SF105A_28' '' } %GIDa_11b1752b_1301_4080_87b8_61785762c695  Port=2
  MotCtrlMotPhaAdv : Outport  RequirementInfo={'linktype_rmi_doors' '0000bb44 (/E-STEER Core/SubSystem Specifications/Application Functions/SF99/SF105A Current Regulator and Voltage Limiter)' '#SF105A_60' 'true' 'REQ: SF105A_60' '' } %GIDa_3db4d37c_18fd_435f_bc3c_57617edd59f1  Port=3
  MotCtrlMotVltgDax : Outport  RequirementInfo={'linktype_rmi_doors' '0000bb44 (/E-STEER Core/SubSystem Specifications/Application Functions/SF99/SF105A Current Regulator and Voltage Limiter)' '#SF105A_63' 'true' 'REQ: SF105A_63' '' } %GIDa_eb8d3c57_82f5_4307_9bf0_3d164d057d5b  Port=4
  MotCtrlMotVltgQax : Outport  RequirementInfo={'linktype_rmi_doors' '0000bb44 (/E-STEER Core/SubSystem Specifications/Application Functions/SF99/SF105A Current Regulator and Voltage Limiter)' '#SF105A_62' 'true' 'REQ: SF105A_62' '' } %GIDa_ac3c9ce4_7911_4bdc_be75_c8defcf1b6a7  Port=5
  wires:
  MotCtrlMotCurrDaxCmd/1 -> MotCurrRegVltgLimrPer1/8(MotCtrlMotCurrDaxCmd)
  MotCtrlBrdgVltg/1 -> MotCurrRegVltgLimrPer1/1(MotCtrlBrdgVltg)
  MotCtrlMotCurrQaxCoggCmd/1 -> MotCurrRegVltgLimrPer1/10(MotCtrlMotCurrQaxCoggCmd)
  MotCtrlMotAgElecDly/1 -> MotCurrRegVltgLimrPer1/5(MotCtrlMotAgElecDly)
  MotCtrlMotCurrDaxMax/1 -> MotCurrRegVltgLimrPer1/7(MotCtrlMotCurrDaxMax)
  MotCtrlMotCurrQax/1 -> MotCurrRegVltgLimrPer1/9(MotCtrlMotCurrQax)
  MotCtrlCurrMeasLoaMtgtnEna/1 -> MotCurrRegVltgLimrPer1/2(MotCtrlCurrMeasLoaMtgtnEna)
  MotCtrlMotCurrDax/1 -> MotCurrRegVltgLimrPer1/6(MotCtrlMotCurrDax)
  MotCtrlMotCurrQaxCmd/1 -> MotCurrRegVltgLimrPer1/11(MotCtrlMotCurrQaxCmd)
  MotCtrlMotCurrQaxRplCmd/1 -> MotCurrRegVltgLimrPer1/12(MotCtrlMotCurrQaxRplCmd)
  MotCtrlMotDampgDax/1 -> MotCurrRegVltgLimrPer1/13(MotCtrlMotDampgDax)
  MotCtrlMotDampgQax/1 -> MotCurrRegVltgLimrPer1/14(MotCtrlMotDampgQax)
  MotCtrlMotReacncDax/1 -> MotCurrRegVltgLimrPer1/15(MotCtrlMotReacncDax)
  MotCtrlMotReacncQax/1 -> MotCurrRegVltgLimrPer1/16(MotCtrlMotReacncQax)
  MotCtrlMotIntglGainDax/1 -> MotCurrRegVltgLimrPer1/17(MotCtrlMotIntglGainDax)
  MotCtrlMotIntglGainQax/1 -> MotCurrRegVltgLimrPer1/18(MotCtrlMotIntglGainQax)
  MotCtrlMotPropGainDax/1 -> MotCurrRegVltgLimrPer1/19(MotCtrlMotPropGainDax)
  MotCtrlMotPropGainQax/1 -> MotCurrRegVltgLimrPer1/20(MotCtrlMotPropGainQax)
  MotCtrlMotVltgDaxFf/1 -> MotCurrRegVltgLimrPer1/21(MotCtrlMotVltgDaxFf)
  MotCtrlMotVltgQaxFf/1 -> MotCurrRegVltgLimrPer1/22(MotCtrlMotVltgQaxFf)
  MotCurrRegVltgLimrPer1/1(MotCtrlMotCurrQaxCmdFinal) -> MotCtrlMotCurrQaxCmdFinal/1
  MotCurrRegVltgLimrPer1/2(MotCtrlMotModlnIdx) -> MotCtrlMotModlnIdx/1
  MotCurrRegVltgLimrPer1/3(MotCtrlMotPhaAdv) -> MotCtrlMotPhaAdv/1
  MotCurrRegVltgLimrPer1/4(MotCtrlMotVltgDax) -> MotCtrlMotVltgDax/1
  MotCurrRegVltgLimrPer1/5(MotCtrlMotVltgQax) -> MotCtrlMotVltgQax/1
  call_MotCurrRegVltgLimrPer1/1 -> MotCurrRegVltgLimrPer1/Trigger
  MotCtrlIvtrLoaMtgtnEna/1 -> MotCurrRegVltgLimrPer1/3(MotCtrlIvtrLoaMtgtnEna)
  MotCtrlSysSt/1 -> MotCurrRegVltgLimrPer1/23(MotCtrlSysSt)
  call_MotCurrRegVltgInit1/1 -> MotCurrRegVltgLimrInit1/Trigger
  MotCtrlMotBackEmfVltg/1 -> MotCurrRegVltgLimrPer1/24(MotCtrlMotBackEmfVltg)
  MotCtrlMotREstimd/1 -> MotCurrRegVltgLimrPer1/25("MotCtrlMotREstimd ")
  MotCtrlMotInduDaxEstimdIvs/1 -> MotCurrRegVltgLimrPer1/26(MotCtrlMotInduDaxEstimdIvs)
  MotCtrlMotInduQaxEstimdIvs/1 -> MotCurrRegVltgLimrPer1/27(MotCtrlMotInduQaxEstimdIvs)
  MotCtrlDualEcuMotCtrlMtgtnEna/1 -> MotCurrRegVltgLimrPer1/4(MotCtrlDualEcuMotCtrlMtgtnEna)

== system SF105A_MotCurrRegVltgLimr/MotCurrRegVltgLimr/CopyRight2 ==

== system SF105A_MotCurrRegVltgLimr/MotCurrRegVltgLimr/MotCurrRegVltgLimrInit1 ==
  function : TriggerPort  TriggerType=function-call
  Constant : Constant  RequirementInfo={'linktype_rmi_doors' '0000bb44 (/E-STEER Core/SubSystem Specifications/Application Functions/SF99/SF105A Current Regulator and Voltage Limiter)' '#SF105A_141' 'true' 'REQ: SF105A_141' '' } %GIDa_11128f3d_f32f_409a_b5cb_fc6065f005cf  OutDataTypeStr=single
  Constant1 : Constant  RequirementInfo={'linktype_rmi_doors' '0000bb44 (/E-STEER Core/SubSystem Specifications/Application Functions/SF99/SF105A Current Regulator and Voltage Limiter)' '#SF105A_141' 'true' 'REQ: SF105A_141' '' } %GIDa_8065204f_b998_4df8_b0ae_ae6693020d34  OutDataTypeStr=single
  Constant2 : Constant  RequirementInfo={'linktype_rmi_doors' '0000bb44 (/E-STEER Core/SubSystem Specifications/Application Functions/SF99/SF105A Current Regulator and Voltage Limiter)' '#SF105A_155' 'true' 'REQ: SF105A_155' '' } %GIDa_c238a597_c539_4ee5_8966_45df3ce9c576  OutDataTypeStr=single
  Constant4 : Constant  RequirementInfo={'linktype_rmi_doors' '0000bb44 (/E-STEER Core/SubSystem Specifications/Application Functions/SF99/SF105A Current Regulator and Voltage Limiter)' '#SF105A_155' 'true' 'REQ: SF105A_155' '' } %GIDa_540d9df7_7d3c_4ab3_9079_d21266d22745  OutDataTypeStr=single
  Constant5 : Constant  RequirementInfo={'linktype_rmi_doors' '0000bb44 (/E-STEER Core/SubSystem Specifications/Application Functions/SF99/SF105A Current Regulator and Voltage Limiter)' '#SF105A_155' 'true' 'REQ: SF105A_155' '' } %GIDa_3bce093a_adf4_4b58_9eb9_1ead50c4137d  OutDataTypeStr=single
  CopyRight2 : Subsystem  Description=|  mask(Copyright Information){none=on}
      | Copyright info block.                                               
      |                                                                     
      | Place copyright information at the top of every subsystem in design.
      mask prompts: none "No parameters"
      mask help: Place copyright information at the top of every subsystem in design.
      mask Display:
      | NxtrConf = 'Nexteer Confidential';
      | 
      | sys = bdroot; %handle for the current model ("system")
      | first = get_param(sys,'Created');
      | if(isempty(first))
      |     first = datestr(now,'yyyy');
      | else
      |     first = first(end-3:end);  %year is last four digits
      | end
      | 
      | last = get_param(sys,'LastModifiedDate');
      | if isempty(last)
      |     last = datestr(now,'yyyy');
      | else
      |     last = last(end-3:end);
      | end
      | 
      | if strcmp(first,last)
      |     fprintf('%s -- Copyright %s Nexteer',NxtrConf,first)
      | else
      |     fprintf('%s -- %s%s- %s Nexteer',NxtrConf,char(169),first,last)
      | end
  Data Store Write : DataStoreWrite  RequirementInfo={'linktype_rmi_doors' '0000bb44 (/E-STEER Core/SubSystem Specifications/Application Functions/SF99/SF105A Current Regulator and Voltage Limiter)' '#SF105A_141' 'true' 'REQ: SF105A_141' '' } %GIDa_339fae29_bd88_40e6_a5f8_62685194cb4e  DataStoreName=AntiWdupCmdScaQax
  Data Store Write1 : DataStoreWrite  RequirementInfo={'linktype_rmi_doors' '0000bb44 (/E-STEER Core/SubSystem Specifications/Application Functions/SF99/SF105A Current Regulator and Voltage Limiter)' '#SF105A_141' 'true' 'REQ: SF105A_141' '' } %GIDa_45e928ad_e824_424e_89b3_5639ae1230e1  DataStoreName=AntiWdupCmdScaDax
  Data Store Write2 : DataStoreWrite  RequirementInfo="{'linktype_rmi_doors' '0000bb44 (/E-STEER Core/SubSystem Specifications/Application Functions/SF99/SF105A Current Regulator and Voltage Limiter)' '#SF105A_155' 'true' 'REQ:  SF105A_155' '' } %GIDa_f70d407e_bed7_462e_b621_3ba5d4f5e334"  DataStoreName=DualEcuLoaScarPrev
  Data Store Write4 : DataStoreWrite  RequirementInfo={'linktype_rmi_doors' '0000bb44 (/E-STEER Core/SubSystem Specifications/Application Functions/SF99/SF105A Current Regulator and Voltage Limiter)' '#SF105A_155' 'true' 'REQ: SF105A_155' '' } %GIDa_ad4a5834_8b04_472e_889e_557ef59e4a22  DataStoreName=CurrLoaScarPrev
  Data Store Write5 : DataStoreWrite  RequirementInfo={'linktype_rmi_doors' '0000bb44 (/E-STEER Core/SubSystem Specifications/Application Functions/SF99/SF105A Current Regulator and Voltage Limiter)' '#SF105A_155' 'true' 'REQ: SF105A_155' '' } %GIDa_a1d3a5d4_c68c_4e65_9c07_621b47011ed7  DataStoreName=IvtrLoaScarPrev
  MotVltgBrdgLpFil : Fil/FilLpInit  Ic=BRDGVLTDFT_VOLT_F32  Ts=ELECGLBPRM_PWMPERDNOMX2_SEC_F32  Freq=MotCurrRegVltgLimrMotVltgBrdgLpFilFrq  StVar=MotVltgBrdgLpFil
  MotVltgQaxFfLpFil : Fil/FilLpInit  Ic=0  Ts=ELECGLBPRM_PWMPERDNOMX2_SEC_F32  Freq=MotCurrRegVltgLimrMotVltgQaxFfLpFilFrq  StVar=MotVltgQaxFfLpFil
  wires:
  Constant/1 -> Data Store Write/1
  Constant1/1 -> Data Store Write1/1
  Constant4/1 -> Data Store Write4/1
  Constant5/1 -> Data Store Write5/1
  Constant2/1 -> Data Store Write2/1
